simulink model "parte1_pert_entrada_discrete"  (R2021b)
settings: Solver=VariableStepAuto  StartTime=0.0  StopTime=6  RelTol=1e-3
values from neighbouring files (symbols this model uses):
  h = 0.03    [parte1_script.m]
  Jm = 1.3475e-6    (= 1.3475e-06)    [parte1_script.m]
  Ke = 0.0159    [parte1_script.m]
  Kf = 0.000001176    (= 1.176e-06)    [parte1_script.m]
  Ki = wn^2 / K1    [parte1_script.m]
  Kp = (2*zeta*wn -alfa)/K1    [parte1_script.m]
  La = 0    [parte1_script.m]
  Ra = 8    [parte1_script.m]
undefined symbols (not defined in the file or in its folder): DiscIntNeverNeededParam
settings Model: Creator=Dylan  LastModifiedBy=Dylan

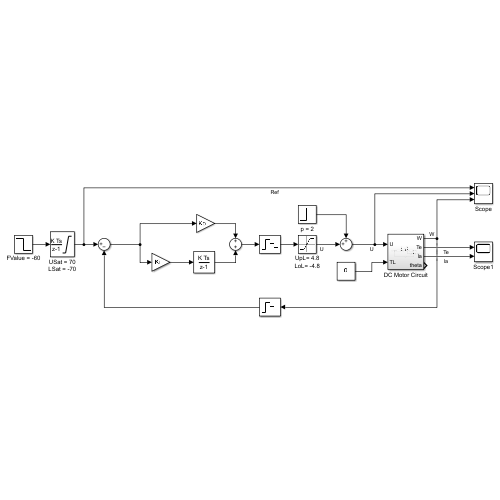
[thumbnail: Simulink's stored preview of the top-level diagram]
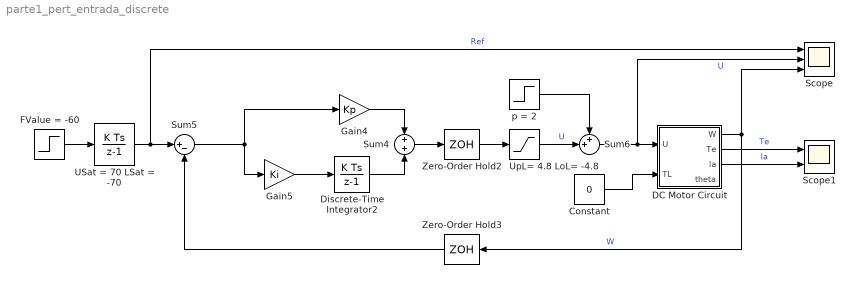
== system parte1_pert_entrada_discrete ==
  Constant : Constant  Value=0
  DC Motor Circuit : Subsystem
  Discrete-Time Integrator2 : DiscreteIntegrator  SampleTime=h  ICPrevOutput=DiscIntNeverNeededParam  ICPrevScaledInput=DiscIntNeverNeededParam
  FValue = -60 : Step  After=-60  SampleTime=0
  Gain4 : Gain  Gain=Kp
  Gain5 : Gain  Gain=Ki
  Scope : Scope  NumInputPorts=3
  Scope1 : Scope  NumInputPorts=2
  Sum4 : Sum  Inputs=+|+
  Sum5 : Sum  Inputs=|+-
  Sum6 : Sum  Inputs=++|
  USat = 70 LSat = -70 : DiscreteIntegrator  SampleTime=h  LimitOutput=on  UpperSaturationLimit=70  LowerSaturationLimit=-70  ICPrevOutput=DiscIntNeverNeededParam  ICPrevScaledInput=DiscIntNeverNeededParam
  UpL= 4.8 LoL= -4.8 : Saturate  UpperLimit=4.8  LowerLimit=-4.8
  Zero-Order Hold2 : ZeroOrderHold  SampleTime=h
  Zero-Order Hold3 : ZeroOrderHold  SampleTime=h
  p = 2 : Step  Time=5  After=2  SampleTime=0
  wires:
  p = 2/1 -> Sum6/1
  USat = 70 LSat = -70/1 -> Scope/1, Sum5/1  "Ref"
  Discrete-Time Integrator2/1 -> Sum4/2
  DC Motor Circuit/2(Te) -> Scope1/1  "Te"
  UpL= 4.8 LoL= -4.8/1 -> Sum6/2  "U"
  FValue = -60/1 -> USat = 70 LSat = -70/1
  DC Motor Circuit/1(W) -> Scope/3, Zero-Order Hold3/1  "W"
  Sum6/1 -> Scope/2, DC Motor Circuit/1(U)  "U"
  Gain4/1 -> Sum4/1
  DC Motor Circuit/3(la) -> Scope1/2  "la"
  Gain5/1 -> Discrete-Time Integrator2/1
  Sum5/1 -> Gain4/1, Gain5/1
  Constant/1 -> DC Motor Circuit/2(TL)
  Sum4/1 -> Zero-Order Hold2/1
  Zero-Order Hold2/1 -> UpL= 4.8 LoL= -4.8/1
  Zero-Order Hold3/1 -> Sum5/2

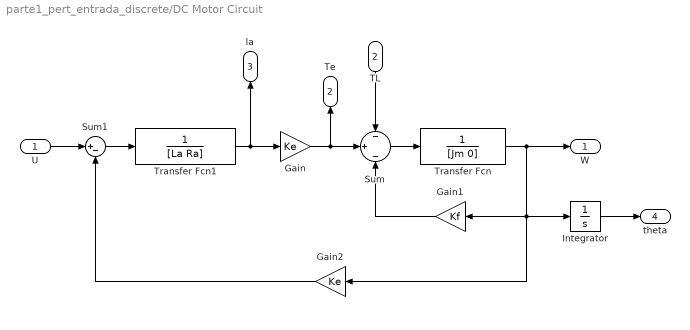
== system parte1_pert_entrada_discrete/DC Motor Circuit ==
  U : Inport
  TL : Inport  Port=2
  Gain : Gain  Gain=Ke
  Gain1 : Gain  Gain=Kf
  Gain2 : Gain  Gain=Ke
  Integrator : Integrator
  Sum : Sum  Inputs=-|+|-
  Sum1 : Sum  Inputs=|+-
  Transfer Fcn : TransferFcn  Denominator=[Jm 0]
  Transfer Fcn1 : TransferFcn  Denominator=[La Ra]
  W : Outport
  Te : Outport  Port=2
  la : Outport  Port=3
  theta : Outport  Port=4
  wires:
  U/1 -> Sum1/1
  Transfer Fcn/1 -> W/1, Gain2/1, Integrator/1, Gain1/1
  Transfer Fcn1/1 -> la/1, Gain/1
  Gain2/1 -> Sum1/2
  Sum/1 -> Transfer Fcn/1
  Gain/1 -> Te/1, Sum/2
  TL/1 -> Sum/1
  Gain1/1 -> Sum/3
  Sum1/1 -> Transfer Fcn1/1
  Integrator/1 -> theta/1
